simulink subsystem "traffic_light_sim_ryg"  (R2024b)
settings: Solver=VariableStepAuto  StartTime=0.0  StopTime=10.0  RelTol=1e-3
settings Model: Creator=nelsenyoung  LastModifiedBy=nelsenyoung

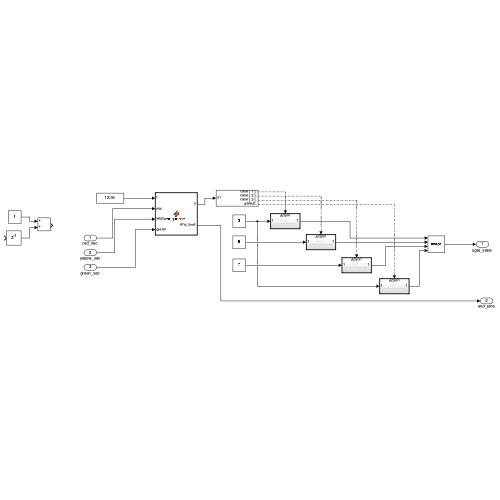
[thumbnail: Simulink's stored preview of the top-level diagram]
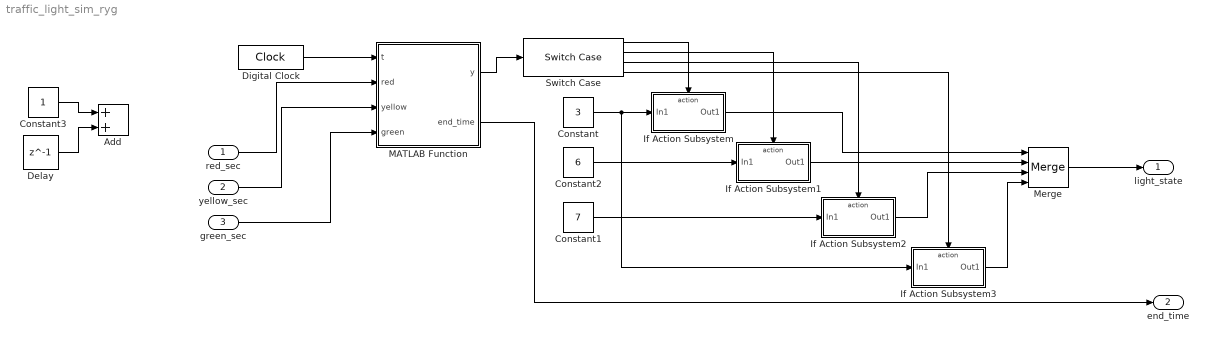
== system traffic_light_sim_ryg ==
  red_sec : Inport
  yellow_sec : Inport  Port=2
  green_sec : Inport  Port=3
  Add : Sum
  Constant : Constant  Value=3
  Constant1 : Constant  Value=7
  Constant2 : Constant  Value=6
  Constant3 : Constant
  Delay : Delay  DelayLength=1
  Digital Clock : DigitalClock  SampleTime=0.1
  If Action Subsystem : Subsystem  TreatAsAtomicUnit=on
  If Action Subsystem1 : Subsystem  TreatAsAtomicUnit=on
  If Action Subsystem2 : Subsystem  TreatAsAtomicUnit=on
  If Action Subsystem3 : Subsystem  TreatAsAtomicUnit=on
  MATLAB Function : MATLAB Function  TreatAsAtomicUnit=on
  Merge : Merge  Inputs=4
  Switch Case : SwitchCase  CaseConditions={1,2,3}
  light_state : Outport
  end_time : Outport  Port=2  OutDataTypeStr=double
  wires:
  red_sec/1 -> MATLAB Function/2(red)
  If Action Subsystem1/1(Out1) -> Merge/2
  Merge/1 -> light_state/1
  green_sec/1 -> MATLAB Function/4(green)
  If Action Subsystem2/1(Out1) -> Merge/3
  Switch Case/3 -> If Action Subsystem2/Action
  Constant2/1 -> If Action Subsystem1/1(In1)
  If Action Subsystem/1(Out1) -> Merge/1
  Switch Case/2 -> If Action Subsystem1/Action
  Switch Case/1 -> If Action Subsystem/Action
  Switch Case/4 -> If Action Subsystem3/Action
  Constant1/1 -> If Action Subsystem2/1(In1)
  yellow_sec/1 -> MATLAB Function/3(yellow)
  Constant/1 -> If Action Subsystem/1(In1), If Action Subsystem3/1(In1)
  Digital Clock/1 -> MATLAB Function/1(t)
  If Action Subsystem3/1(Out1) -> Merge/4
  MATLAB Function/1(y) -> Switch Case/1
  MATLAB Function/2(end_time) -> end_time/1
  Delay/1 -> Add/2
  Constant3/1 -> Add/1

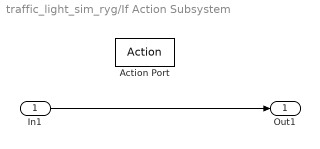
== system traffic_light_sim_ryg/If Action Subsystem ==
  In1 : Inport
  Action Port : ActionPort
  Out1 : Outport
  wires:
  In1/1 -> Out1/1

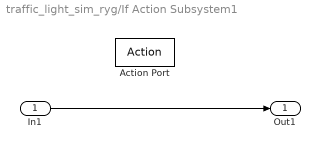
== system traffic_light_sim_ryg/If Action Subsystem1 ==
  In1 : Inport
  Action Port : ActionPort
  Out1 : Outport
  wires:
  In1/1 -> Out1/1

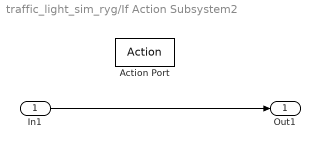
== system traffic_light_sim_ryg/If Action Subsystem2 ==
  In1 : Inport
  Action Port : ActionPort
  Out1 : Outport
  wires:
  In1/1 -> Out1/1

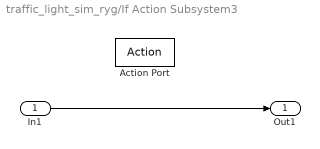
== system traffic_light_sim_ryg/If Action Subsystem3 ==
  In1 : Inport
  Action Port : ActionPort
  Out1 : Outport
  wires:
  In1/1 -> Out1/1

== matlab function traffic_light_sim_ryg/MATLAB Function ==
  data: t input; y output; red input; yellow input; green input; end_time output
function [y,end_time] = sequence(t, red, yellow, green)
    % Define the repeating time pattern
    cycleTime = red + yellow + green;
    T = mod(t, cycleTime); % Reset every 25 seconds
    if T == 0
        y = 3;
        end_time = 0;
    elseif T <= red
        y = 1;
        end_time = red - T;
    elseif T <= red + green
        y = 2;
        end_time = (red + green) - T;
    elseif T <= cycleTime
        y = 3;
        end_time = cycleTime - T;
    else
        y = 1;
        end_time = 0;
    end
end
